simulink model "controllerCodeGenerationWrapper"  (R2022a)
settings: configuration reference "ControllerCodeGenerationConfigurationSet" (kept outside this file)
model workspace (MAT data in the model file):
  CONTROLLER_CLIENT_DEVICE_ID_LIST_NVM_ADDRESS_AS_UINT32 = Simulink.Parameter
  CONTROLLER_CLIENT_DEVICE_ID_LIST_NVM_ADDRESS_AS_UINT32.Value = 1234
  CONTROLLER_CLIENT_DEVICE_ID_LIST_NVM_ADDRESS_AS_UINT32.DataType = 'uint32'
  CONTROLLER_CLIENT_DEVICE_ID_LIST_NVM_ADDRESS_AS_UINT32.Complexity = 'real'
  CONTROLLER_CLIENT_DEVICE_ID_LIST_NVM_ADDRESS_AS_UINT32.Dimensions = [1 1]
  CONTROLLER_FAULT_LOG_NVM_ADDRESS_AS_UINT32 = Simulink.Parameter
  CONTROLLER_FAULT_LOG_NVM_ADDRESS_AS_UINT32.Value = 3456
  CONTROLLER_FAULT_LOG_NVM_ADDRESS_AS_UINT32.DataType = 'uint32'
  CONTROLLER_FAULT_LOG_NVM_ADDRESS_AS_UINT32.Complexity = 'real'
  CONTROLLER_FAULT_LOG_NVM_ADDRESS_AS_UINT32.Dimensions = [1 1]
undefined symbols (not defined in the file): DEFAULT_CLIENT_DEVICE_ID_LIST, DEFAULT_MEASUREMENT_MSG_BUS_TYPE, PER_STEP_MAXIMUM_MESSAGES_TO_PROCESS
settings Model: DataDictionary=controllerTargetSpecificData.sldd  EnableAccessToBaseWorkspace=off  Creator=The MathWorks, Inc.  LastModifiedBy=The MathWorks, Inc.
settings ConfigSetRef: SourceName=ControllerCodeGenerationConfigurationSet

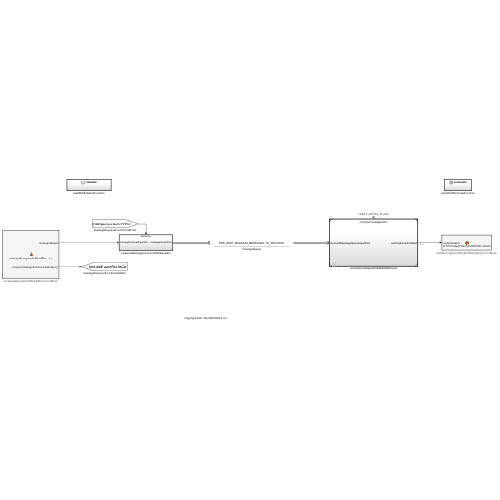
[thumbnail: Simulink's stored preview of the top-level diagram]
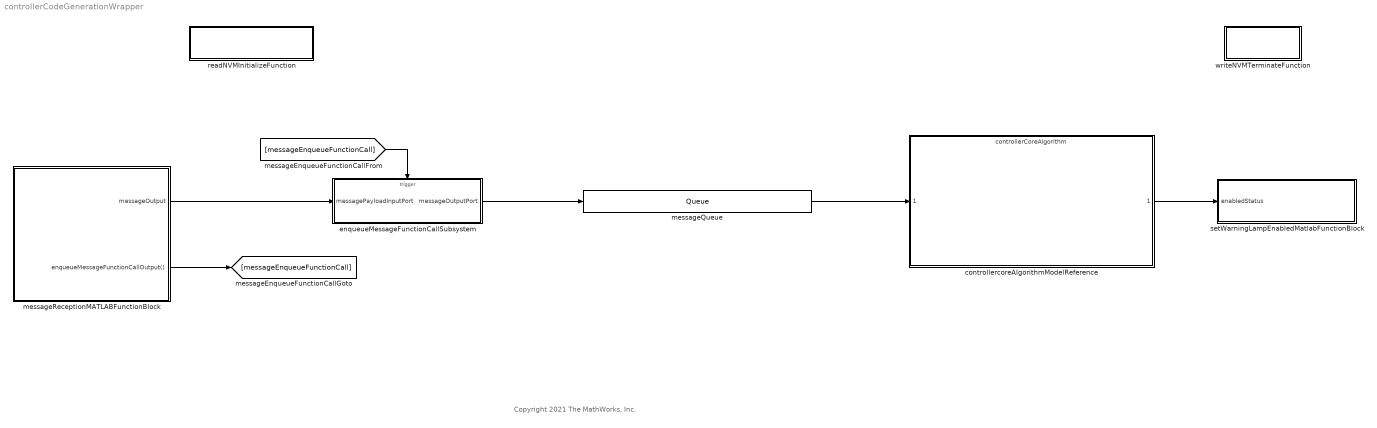
== system controllerCodeGenerationWrapper ==
  note: Copyright 2021 The MathWorks, Inc.
  controllercoreAlgorithmModelReference : ModelReference  InputPortMessageModes=m  ModelNameDialog=controllerCoreAlgorithm  UsingDefaultArgumentValue=0  SimulationMode=Normal  ModelReferenceVersion=4.0
  enqueueMessageFunctionCallSubsystem : Subsystem  TreatAsAtomicUnit=on
  messageQueue : Queue  InputPortMessageModes=m  OutputPortMessageModes=m  OverwriteOldest=on  Capacity=PER_STEP_MAXIMUM_MESSAGES_TO_PROCESS  QueueType=LIFO
  messageReceptionMATLABFunctionBlock : MATLAB Function  TreatAsAtomicUnit=on
  readNVMInitializeFunction : Subsystem  TreatAsAtomicUnit=on
  setWarningLampEnabledMatlabFunctionBlock : MATLAB Function  TreatAsAtomicUnit=on
  writeNVMTerminateFunction : Subsystem  TreatAsAtomicUnit=on
  wires:
  controllercoreAlgorithmModelReference/1 -> setWarningLampEnabledMatlabFunctionBlock/1(enabledStatus)
  messageReceptionMATLABFunctionBlock/1(messageOutput) -> enqueueMessageFunctionCallSubsystem/1(messagePayloadInputPort)
  messageReceptionMATLABFunctionBlock/2(enqueueMessageFunctionCallOutput()) -> [messageEnqueueFunctionCall]
  enqueueMessageFunctionCallSubsystem/1(messageOutputPort) -> messageQueue/1
  [messageEnqueueFunctionCall] -> enqueueMessageFunctionCallSubsystem/Trigger
  messageQueue/1 -> controllercoreAlgorithmModelReference/1

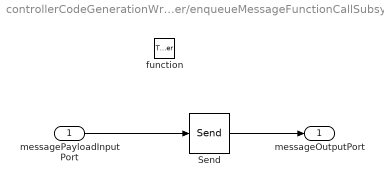
== system controllerCodeGenerationWrapper/enqueueMessageFunctionCallSubsystem ==
  messagePayloadInputPort : Inport
  function : TriggerPort  TriggerType=function-call  VariantControl=(inherit)
  Send : Send  OutputPortMessageModes=m
  messageOutputPort : Outport
  wires:
  Send/1 -> messageOutputPort/1
  messagePayloadInputPort/1 -> Send/1

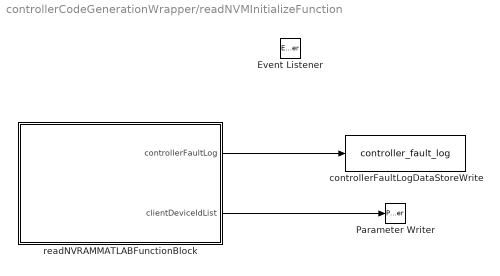
== system controllerCodeGenerationWrapper/readNVMInitializeFunction ==
  Event Listener : EventListener  DisableCoverage=on  EventName=reset
  Parameter Writer : ParameterWriter  ParameterOwnerBlock=../../controllercoreAlgorithmModelReference  ParameterName=CLIENT_DEVICE_ID_LIST  ParameterInternalName=CLIENT_DEVICE_ID_LIST
  controllerFaultLogDataStoreWrite : DataStoreWrite  DataStoreName=controller_fault_log  IndexOptions=Index vector (dialog)  Indices=1  OutputSizes=1
  readNVRAMMATLABFunctionBlock : MATLAB Function  TreatAsAtomicUnit=on
  wires:
  readNVRAMMATLABFunctionBlock/2(clientDeviceIdList) -> Parameter Writer/1
  readNVRAMMATLABFunctionBlock/1(controllerFaultLog) -> controllerFaultLogDataStoreWrite/1

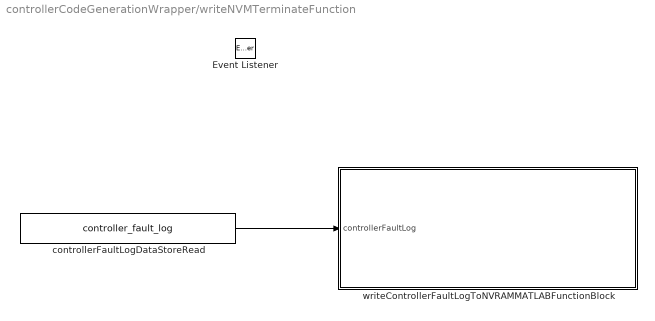
== system controllerCodeGenerationWrapper/writeNVMTerminateFunction ==
  Event Listener : EventListener  DisableCoverage=on  EventType=Terminate  EventName=reset
  controllerFaultLogDataStoreRead : DataStoreRead  DataStoreName=controller_fault_log  IndexOptions=Index vector (dialog)  Indices=1  OutputSizes=1
  writeControllerFaultLogToNVRAMMATLABFunctionBlock : MATLAB Function  TreatAsAtomicUnit=on
  wires:
  controllerFaultLogDataStoreRead/1 -> writeControllerFaultLogToNVRAMMATLABFunctionBlock/1(controllerFaultLog)

== matlab function controllerCodeGenerationWrapper/readNVMInitializeFunction/readNVRAMMATLABFunctionBlock ==
  data: controllerFaultLog output Bus: ControllerFaultLogEntryBusType size=[ 10, 1 ]; clientDeviceIdList output Bus: DeviceIDBusType size=[ 4, 1 ]; CONTROLLER_CLIENT_DEVICE_ID_LIST_NVM_ADDRESS_AS_UINT32 parameter; CONTROLLER_FAULT_LOG_NVM_ADDRESS_AS_UINT32 parameter; DEFAULT_CLIENT_DEVICE_ID_LIST parameter
function [ controllerFaultLog, clientDeviceIdList ] = readNVRAMMATLABFunction( CONTROLLER_CLIENT_DEVICE_ID_LIST_NVM_ADDRESS_AS_UINT32, CONTROLLER_FAULT_LOG_NVM_ADDRESS_AS_UINT32, DEFAULT_CLIENT_DEVICE_ID_LIST )

coder.extrinsic( 'warning' );

controllerFaultLog = ...
    repmat( controllerFaultLogEntryBusTypeDefaultConstructor( ), 10, 1 );

clientDeviceIdList = DEFAULT_CLIENT_DEVICE_ID_LIST;

if( coder.target( 'Rtw' ) )

    clientDeviceIdList = ...    
    ControllerTargetSpecificCodeExternalDependency.nvmReadMatlabWrapper( CONTROLLER_CLIENT_DEVICE_ID_LIST_NVM_ADDRESS_AS_UINT32, clientDeviceIdList );

controllerFaultLog = ...
    ControllerTargetSpecificCodeExternalDependency.nvmReadMatlabWrapper( CONTROLLER_FAULT_LOG_NVM_ADDRESS_AS_UINT32, controllerFaultLog );

else
    warning( 'This block is only used for code-generation.' );    
end

return;

end

== matlab function controllerCodeGenerationWrapper/writeNVMTerminateFunction/writeControllerFaultLogToNVRAMMATLABFunctionBlock ==
  data: CONTROLLER_FAULT_LOG_NVM_ADDRESS_AS_UINT32 parameter; controllerFaultLog input Bus: ControllerFaultLogEntryBusType
function  writeControllerFaultLogToNVRAMMATLABFunction(CONTROLLER_FAULT_LOG_NVM_ADDRESS_AS_UINT32, controllerFaultLog)

coder.extrinsic( 'warning' );

if( coder.target( 'Rtw' ) )

    ControllerTargetSpecificCodeExternalDependency.nvmWriteMatlabWrapper( CONTROLLER_FAULT_LOG_NVM_ADDRESS_AS_UINT32, controllerFaultLog );

else
    warning( 'This block is only used for code-generation.' );
end

return;

end

== matlab function controllerCodeGenerationWrapper/setWarningLampEnabledMatlabFunctionBlock ==
  data: enabledStatus input
function setWarningLampEnabledMatlabFunction( enabledStatus )

coder.extrinsic( 'warning' );

if( coder.target( 'Rtw' ) )

    ControllerTargetSpecificCodeExternalDependency.setWarningLampEnabledMatlabWrapper( enabledStatus );

else
    warning( 'This block is only used for code-generation.' );
end

return;
end

== matlab function controllerCodeGenerationWrapper/messageReceptionMATLABFunctionBlock ==
  data: messageOutput output Bus: MeasurementMsgBusType; DEFAULT_MEASUREMENT_MSG_BUS_TYPE parameter; PER_STEP_MAXIMUM_MESSAGES_TO_PROCESS parameter
  events: enqueueMessageFunctionCallOutput output FUNCTION_CALL_EVENT
 function messageOutput   = messageReceptionMATLABFunction( DEFAULT_MEASUREMENT_MSG_BUS_TYPE, PER_STEP_MAXIMUM_MESSAGES_TO_PROCESS )

coder.extrinsic( 'warning' );

messageOutput = DEFAULT_MEASUREMENT_MSG_BUS_TYPE;

if( coder.target( 'Rtw' ) )

    for processedMessageQuantity = 1 : PER_STEP_MAXIMUM_MESSAGES_TO_PROCESS

        messageOutput = measurementMsgBusTypeDefaultConstructor( );

        messageByteQuantityAsSizeT = coder.opaque( 'size_t', '0' );

        messageByteQuantityAsSizeT = coder.ceval( 'sizeof', messageOutput );

        receptionQueueMessageByteQuantityAsUint32 = ...
            ControllerTargetSpecificCodeExternalDependency.getReceptionQueueMessageByteQuantityMatlabWrapper( );

        messageByteQuantityAsUint32 = ...
            cast( messageByteQuantityAsSizeT, 'like', receptionQueueMessageByteQuantityAsUint32 );

        messageReceived = ...
            ( messageByteQuantityAsUint32 < receptionQueueMessageByteQuantityAsUint32 );

        if( true == messageReceived )

            messageOutput = ...
                ControllerTargetSpecificCodeExternalDependency.getMessageBytesMatlabWrapper( messageOutput );

            enqueueMessageFunctionCallOutput( );

        else
            % There are no more messages.
            break;
        end

    end

else
    warning( 'This block is only for code-generation.' );
end

return;

end
